simulink model "ep3_1"  (R2023b)
settings: Solver=VariableStepAuto  StartTime=0.0  StopTime=10.0  RelTol=1e-3
libraries: simulink x1
settings Model: Creator=86186  LastModifiedBy=86186

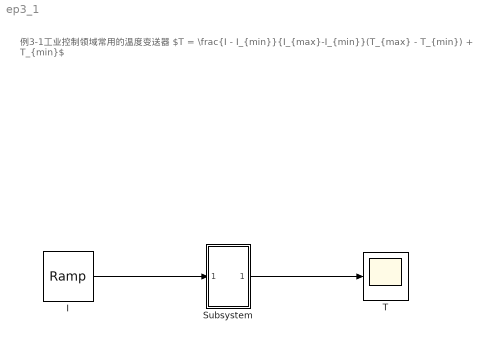
== system ep3_1 ==
  note: 例3-1工业控制领域常用的温度变送器
      | $T = \frac{I - I_{min}}{I_{max}-I_{min}}(T_{max} - T_{min}) + T_{min}$
  I : simulink/Sources/Ramp  slope=1  start=0  InitialOutput=0
  Subsystem : Subsystem  mask{Imin=2, Imax=16, Tmin=-20, Tmax=90}
      mask init:
      | I = 4:0.1:20;
      | Tmax = 40;
      | Tmin = 30;
      | T = (I - 5)./(15-5).*(Tmax-Tmin)+Tmin;
      mask DialogControl ParameterGroupVar Prompt: 参数
      mask Display:
      | plot(I,T);
      | port_label('input', 1, 'I');
      | port_label('output', 1, 'T');
  T : Scope
  wires:
  I/1 -> Subsystem/1(In1)
  Subsystem/1(Out1) -> T/1

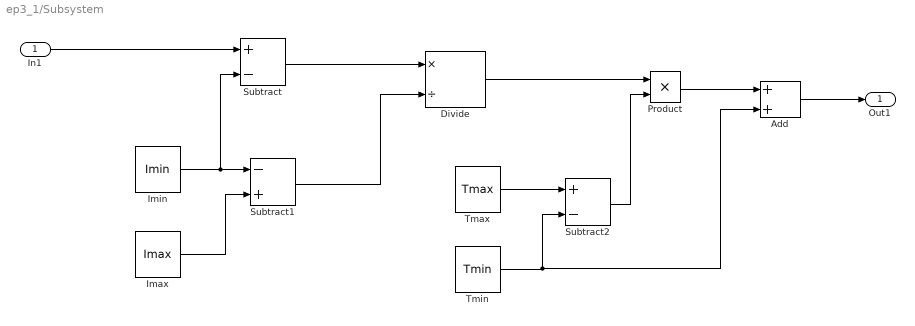
== system ep3_1/Subsystem ==
  In1 : Inport
  Add : Sum
  Divide : Product  Inputs=*/
  Imax : Constant  Value=Imax
  Imin : Constant  Value=Imin
  Product : Product
  Subtract : Sum  Inputs=+-
  Subtract1 : Sum  Inputs=-+
  Subtract2 : Sum  Inputs=+-
  Tmax : Constant  Value=Tmax
  Tmin : Constant  Value=Tmin
  Out1 : Outport
  wires:
  Imin/1 -> Subtract/2, Subtract1/1
  Tmin/1 -> Add/2, Subtract2/2
  Imax/1 -> Subtract1/2
  Subtract/1 -> Divide/1
  Tmax/1 -> Subtract2/1
  Divide/1 -> Product/1
  Subtract1/1 -> Divide/2
  Product/1 -> Add/1
  Subtract2/1 -> Product/2
  In1/1 -> Subtract/1
  Add/1 -> Out1/1
